simulink subsystem "Vehicle1DMinimal_refsub"  (R2020b)
settings: Solver=VariableStepAuto  StartTime=0.0  StopTime=10.0  RelTol=1e-3
undefined symbols (not defined in the file or in its folder): vehicle
libraries: fl_lib x7, nesl_utility x2
settings Model: Creator=isaacito  LastModifiedBy=isaacito

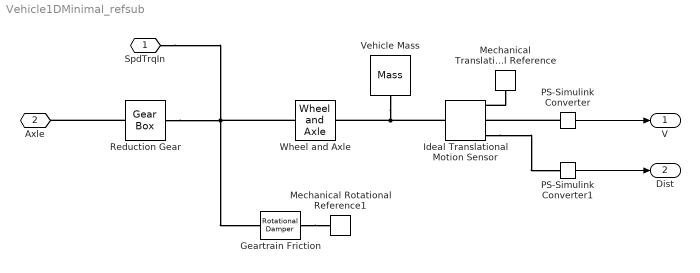
== system Vehicle1DMinimal_refsub ==
  Geartrain Friction : fl_lib/Mechanical/Rotational Elements/Rotational Damper  D=vehicle.geartrainFriction_Nm_per_rpm m*N/rpm  w_specify=off  w_priority=None  w=0 rad/s  w_nominal_specify=off  w_nominal_unit=rad/s  w_nominal_value=1  t_specify=off  t_priority=None  t=0 N*m  t_nominal_specify=off  t_nominal_unit=N*m  t_nominal_value=1
      settings: AttributesFormatString=|
      | %<D>
      | %<D_unit>
  Ideal Translational Motion Sensor : fl_lib/Mechanical/Mechanical Sensors/Ideal Translational Motion Sensor  offset=0 m
      settings: AttributesFormatString=Initial: %<offset> %<offset_unit>
  Mechanical Rotational Reference1 : fl_lib/Mechanical/Rotational Elements/Mechanical Rotational Reference
  Mechanical Translational Reference : fl_lib/Mechanical/Translational Elements/Mechanical Translational Reference
  PS-Simulink Converter : nesl_utility/PS-Simulink Converter  PhysicalDomain=network_engine_domain  SubClassName=ps_output  LeftPortType=input  RightPortType=output  PseudoPeriodic=off  Frequencies=[]  Unit=km/hr  AffineConversion=off
  PS-Simulink Converter1 : nesl_utility/PS-Simulink Converter  PhysicalDomain=network_engine_domain  SubClassName=ps_output  LeftPortType=input  RightPortType=output  PseudoPeriodic=off  Frequencies=[]  Unit=km  AffineConversion=off
  Reduction Gear : fl_lib/Mechanical/Mechanisms/Gear Box  ratio=vehicle.reducerGearRatio_1  t_in_specify=off  t_in_priority=None  t_in=0 N*m  t_in_nominal_specify=off  t_in_nominal_unit=N*m  t_in_nominal_value=1  t_out_specify=off  t_out_priority=None  t_out=0 N*m  t_out_nominal_specify=off  t_out_nominal_unit=N*m  t_out_nominal_value=1
      settings: AttributesFormatString=%<ratio>
  Vehicle Mass : fl_lib/Mechanical/Translational Elements/Mass  mass=vehicle.mass_kg kg  num_ports=foundation.enum.numPorts2.one  v_specify=on  v_priority=High  v=initial.vehicleSpeed_kph km/hr  v_nominal_specify=off  v_nominal_unit=m/s  v_nominal_value=1  f_specify=off  f_priority=None  f=0 N  f_nominal_specify=off  f_nominal_unit=N  f_nominal_value=1
      settings: AttributesFormatString=|
      | %<v> [%<v_unit>]
      | %<mass> [%<mass_unit>]
  Wheel and Axle : fl_lib/Mechanical/Mechanisms/Wheel and Axle  R=vehicle.tireRollingRadius_m m  or=1  t_specify=off  t_priority=None  t=0 N*m  t_nominal_specify=off  t_nominal_unit=N*m  t_nominal_value=1  f_specify=off  f_priority=None  f=0 N  f_nominal_specify=off  f_nominal_unit=N  f_nominal_value=1
      settings: AttributesFormatString=|
      | %<R>
      | %<R_unit>
  SpdTrqIn : PMIOPort  Side=Left
  Axle : PMIOPort  Port=2  Side=Left
  V : Outport
  Dist : Outport  Port=2
  wires:
  PS-Simulink Converter/1 -> V/1
  PS-Simulink Converter1/1 -> Dist/1
  connections:
  Wheel and Axle/LConn1 -- SpdTrqIn/RConn1 -- Geartrain Friction/LConn1 -- Reduction Gear/RConn1
  Ideal Translational Motion Sensor/LConn1 -- Wheel and Axle/RConn1 -- Vehicle Mass/LConn1
  Reduction Gear/LConn1 -- Axle/RConn1
  Geartrain Friction/RConn1 -- Mechanical Rotational Reference1/LConn1
  Ideal Translational Motion Sensor/RConn3 -- PS-Simulink Converter1/LConn1
  Mechanical Translational Reference/LConn1 -- Ideal Translational Motion Sensor/RConn1
  PS-Simulink Converter/LConn1 -- Ideal Translational Motion Sensor/RConn2
